simulink model "brownian_noise_2"  (R2023b)
settings: Solver=VariableStepAuto  StartTime=0.0  StopTime=10.0  RelTol=1e-3
settings Model: Creator=awcm9  LastModifiedBy=awcm9

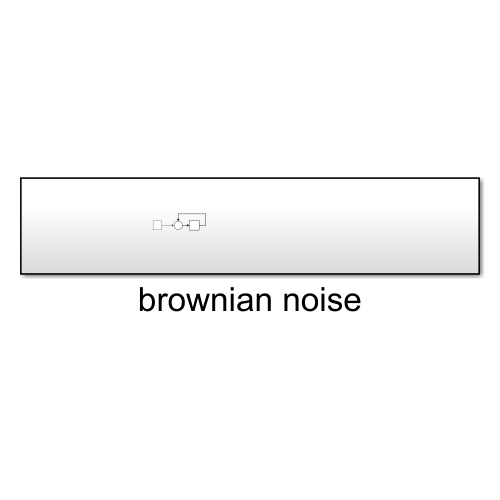
[thumbnail: Simulink's stored preview of the top-level diagram]
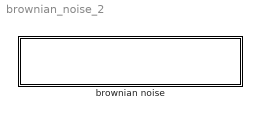
== system brownian_noise_2 ==
  brownian noise : Subsystem

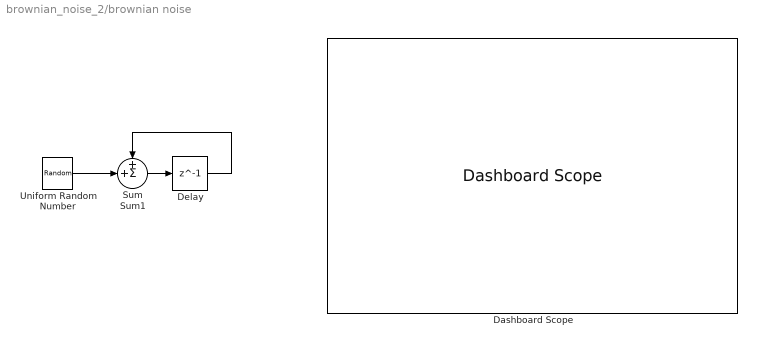
== system brownian_noise_2/brownian noise ==
  " " : Delay  DelayLength=1
  Dashboard Scope : DashboardScope  ShowInitialText=off  TimeSpan=15  Ymin=-30  Ymax=30  ScaleAtStop=off
  Delay : Delay  DelayLength=1
  Sum : Sum  Inputs=++|
  Sum1 : Sum  Inputs=+|
  Uniform Random Number : UniformRandomNumber  SampleTime=1
  wires:
  Uniform Random Number/1 -> Sum/2
  Delay/1 -> Sum1/1
  Sum/1 -> Delay/1
  Sum1/1 -> " "/1
  " "/1 -> Sum/1
